simulink model "PWM_constant"  (R2020a)
settings: Solver=VariableStepAuto  StartTime=0.0  StopTime=0.2  RelTol=1e-3
libraries: simulink x1, powerlib_meascontrol x1
settings Model: Creator=Naeem Mohammad  LastModifiedBy=Naeem Mohammad

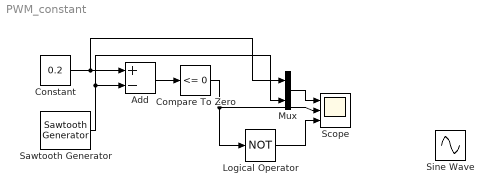
== system PWM_constant ==
  Add : Sum  Inputs=+-
  Compare To Zero : simulink/Logic and Bit Operations/Compare To Zero  relop=<=  OutDataTypeStr=boolean
  Constant : Constant  Value=0.2
  Logical Operator : Logic  Operator=NOT  AllPortsSameDT=off  OutDataTypeStr=boolean
  Mux : Mux  Inputs=2
  Sawtooth Generator : powerlib_meascontrol/Pulse & Signal Generators/Sawtooth Generator  Freq=60  Phase=180  Ts=0
  Scope : Scope  NumInputPorts=3
  Sine Wave : Sin  Amplitude=0.75  Frequency=60  SampleTime=0
  wires:
  Add/1 -> Compare To Zero/1
  Constant/1 -> Add/1, Mux/1
  Sawtooth Generator/1 -> Mux/2, Add/2
  Compare To Zero/1 -> Scope/2, Logical Operator/1
  Logical Operator/1 -> Scope/3
  Mux/1 -> Scope/1
